simulink model "sm_forklift"  (R2021b)
settings: Solver=ode15s  StartTime=0.0  StopTime=53  MaxStep=1e-2  RelTol=1e-3  AbsTol=1e-3  EnableMultiTasking=on
model workspace: external: MATLAB File sm_forklift_parameters.m (data not in the file)
values from neighbouring files (symbols this model uses):
  g = 9.8    [sm_forklift_parameters.m]
undefined symbols (not defined in the file or in its folder): backRest, box, bump, chassis, fork, infPlane, main_mast, pulley, smiData, tire, top_mast, wheel, X, Y, Z
libraries: sm_lib x1413, nesl_utility x83, fl_lib x23, sm_backhoe_lib x6, SignalEditorBlockLib x1
(part 10 of 24)

== system sm_forklift/Warehouse/Racks/Rack 2/Rack End  ==
  Rack_AngleBrace_21_RIGID : Subsystem
  Rack_AngleBrace_22_RIGID : Subsystem
  Rack_AngleBrace_23_RIGID : Subsystem
  Rack_AngleBrace_24_RIGID : Subsystem
  Rack_AngleBrace_25_RIGID : Subsystem
  Rack_Leg_10_RIGID : Subsystem
  Rack_Leg_9_RIGID : Subsystem
  Rack_ShelfEnd_29_RIGID : Subsystem
  Rack_ShelfEnd_30_RIGID : Subsystem
  Rack_ShelfEnd_31_RIGID : Subsystem
  Rack_ShelfEnd_32_RIGID : Subsystem
  Rack_ShelfEnd_33_RIGID : Subsystem
  Rack_ShelfEnd_34_RIGID : Subsystem
  Rack_ShelfEnd_35_RIGID : Subsystem
  Conn1 : PMIOPort  Side=Left
  connections:
  Conn1/RConn1 -- Rack_ShelfEnd_29_RIGID/LConn2
  Rack_Leg_10_RIGID/LConn1 -- Rack_AngleBrace_25_RIGID/LConn1 -- Rack_AngleBrace_24_RIGID/LConn1 -- Rack_AngleBrace_23_RIGID/LConn1 -- Rack_AngleBrace_22_RIGID/LConn1 -- Rack_ShelfEnd_35_RIGID/LConn1 -- Rack_ShelfEnd_34_RIGID/LConn1 -- Rack_ShelfEnd_33_RIGID/LConn1 -- Rack_ShelfEnd_32_RIGID/LConn1 -- Rack_ShelfEnd_31_RIGID/LConn1 -- Rack_ShelfEnd_29_RIGID/LConn1 -- Rack_AngleBrace_21_RIGID/LConn1 -- Rack_ShelfEnd_30_RIGID/LConn1 -- Rack_Leg_9_RIGID/LConn1

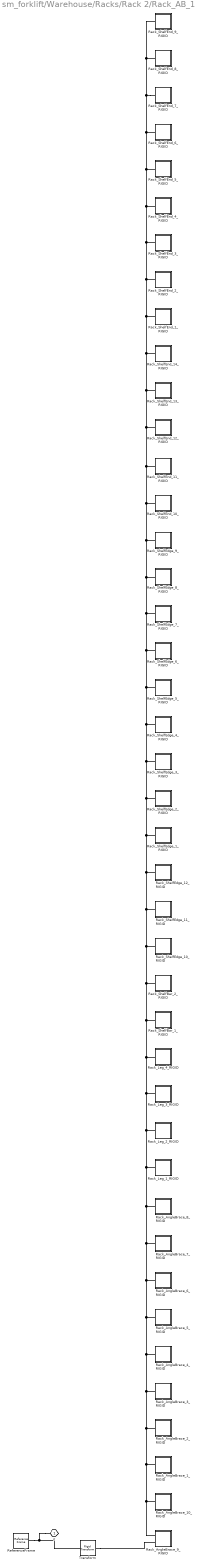
== system sm_forklift/Warehouse/Racks/Rack 2/Rack_AB_1 ==
  Rack_AngleBrace_10_RIGID : Subsystem
  Rack_AngleBrace_1_RIGID : Subsystem
  Rack_AngleBrace_2_RIGID : Subsystem
  Rack_AngleBrace_3_RIGID : Subsystem
  Rack_AngleBrace_4_RIGID : Subsystem
  Rack_AngleBrace_5_RIGID : Subsystem
  Rack_AngleBrace_6_RIGID : Subsystem
  Rack_AngleBrace_7_RIGID : Subsystem
  Rack_AngleBrace_8_RIGID : Subsystem
  Rack_AngleBrace_9_RIGID : Subsystem
  Rack_Leg_1_RIGID : Subsystem
  Rack_Leg_2_RIGID : Subsystem
  Rack_Leg_3_RIGID : Subsystem
  Rack_Leg_4_RIGID : Subsystem
  Rack_ShelfBar_1_RIGID : Subsystem
  Rack_ShelfBar_2_RIGID : Subsystem
  Rack_ShelfEdge_10_RIGID : Subsystem
  Rack_ShelfEdge_11_RIGID : Subsystem
  Rack_ShelfEdge_12_RIGID : Subsystem
  Rack_ShelfEdge_1_RIGID : Subsystem
  Rack_ShelfEdge_2_RIGID : Subsystem
  Rack_ShelfEdge_3_RIGID : Subsystem
  Rack_ShelfEdge_4_RIGID : Subsystem
  Rack_ShelfEdge_5_RIGID : Subsystem
  Rack_ShelfEdge_6_RIGID : Subsystem
  Rack_ShelfEdge_7_RIGID : Subsystem
  Rack_ShelfEdge_8_RIGID : Subsystem
  Rack_ShelfEdge_9_RIGID : Subsystem
  Rack_ShelfEnd_10_RIGID : Subsystem
  Rack_ShelfEnd_11_RIGID : Subsystem
  Rack_ShelfEnd_12_RIGID : Subsystem
  Rack_ShelfEnd_13_RIGID : Subsystem
  Rack_ShelfEnd_14_RIGID : Subsystem
  Rack_ShelfEnd_1_RIGID : Subsystem
  Rack_ShelfEnd_2_RIGID : Subsystem
  Rack_ShelfEnd_3_RIGID : Subsystem
  Rack_ShelfEnd_4_RIGID : Subsystem
  Rack_ShelfEnd_5_RIGID : Subsystem
  Rack_ShelfEnd_6_RIGID : Subsystem
  Rack_ShelfEnd_7_RIGID : Subsystem
  Rack_ShelfEnd_8_RIGID : Subsystem
  Rack_ShelfEnd_9_RIGID : Subsystem
  ReferenceFrame : sm_lib/Frames and Transforms/Reference Frame
  Transform : sm_lib/Frames and Transforms/Rigid Transform  TranslationMethod=Cartesian  TranslationStandardOffset=0  TranslationLengthUnit=m  TranslationStandardAxis=+Z  TranslationCartesianOffset=smiData.RigidTransform(197).translation  TranslationROffset=0  TranslationROffsetUnits=m  TranslationZOffset=0  TranslationZOffsetUnits=m  TranslationThetaOffset=0  TranslationThetaOffsetUnits=deg  RotationMethod=ArbitraryAxis  RotationAngleUnits=rad  RotationStandardAxis=+Z  RotationAngle=smiData.RigidTransform(197).angle  RotationArbitraryAxis=smiData.RigidTransform(197).axis  FollAlignAxisA=+X  BaseAlignAxisA=+Y  FollAlignAxisB=+Y  BaseAlignAxisB=+Z  RotationSequenceAxes=FollowerAxes  RotationSequence=XYX  RotationSequenceAngles=[0 0 0]  RotationSequenceAnglesUnits=deg  RotationMatrix=[1 0 0; 0 1 0; 0 0 1]
  F : PMIOPort  Side=Left
  connections:
  F/RConn1 -- Transform/LConn1 -- ReferenceFrame/RConn1
  Transform/RConn1 -- Rack_AngleBrace_9_RIGID/LConn2
  Rack_ShelfEnd_7_RIGID/LConn1 -- Rack_ShelfEnd_6_RIGID/LConn1 -- Rack_ShelfEnd_5_RIGID/LConn1 -- Rack_ShelfEnd_4_RIGID/LConn1 -- Rack_ShelfEnd_3_RIGID/LConn1 -- Rack_ShelfEnd_2_RIGID/LConn1 -- Rack_ShelfEnd_1_RIGID/LConn1 -- Rack_ShelfEnd_14_RIGID/LConn1 -- Rack_ShelfEnd_13_RIGID/LConn1 -- Rack_ShelfEnd_12_RIGID/LConn1 -- Rack_ShelfEnd_11_RIGID/LConn1 -- Rack_ShelfEnd_10_RIGID/LConn1 -- Rack_ShelfEdge_9_RIGID/LConn1 -- Rack_ShelfEdge_8_RIGID/LConn1 -- Rack_ShelfEdge_7_RIGID/LConn1 -- Rack_ShelfEdge_6_RIGID/LConn1 -- Rack_ShelfEdge_5_RIGID/LConn1 -- Rack_ShelfEdge_4_RIGID/LConn1 -- Rack_ShelfEdge_3_RIGID/LConn1 -- Rack_ShelfEdge_2_RIGID/LConn1 -- Rack_ShelfEdge_1_RIGID/LConn1 -- Rack_ShelfEdge_12_RIGID/LConn1 -- Rack_ShelfEdge_11_RIGID/LConn1 -- Rack_ShelfEdge_10_RIGID/LConn1 -- Rack_ShelfBar_2_RIGID/LConn1 -- Rack_ShelfBar_1_RIGID/LConn1 -- Rack_Leg_4_RIGID/LConn1 -- Rack_Leg_3_RIGID/LConn1 -- Rack_Leg_2_RIGID/LConn1 -- Rack_Leg_1_RIGID/LConn1 -- Rack_AngleBrace_8_RIGID/LConn1 -- Rack_AngleBrace_7_RIGID/LConn1 -- Rack_AngleBrace_6_RIGID/LConn1 -- Rack_AngleBrace_5_RIGID/LConn1 -- Rack_AngleBrace_4_RIGID/LConn1 -- Rack_AngleBrace_3_RIGID/LConn1 -- Rack_AngleBrace_2_RIGID/LConn1 -- Rack_AngleBrace_1_RIGID/LConn1 -- Rack_AngleBrace_9_RIGID/LConn1 -- Rack_AngleBrace_10_RIGID/LConn1 -- Rack_ShelfEnd_9_RIGID/LConn1 -- Rack_ShelfEnd_8_RIGID/LConn1

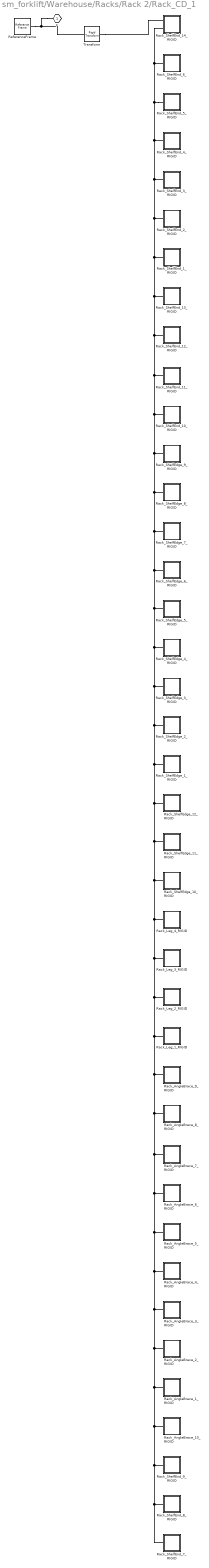
== system sm_forklift/Warehouse/Racks/Rack 2/Rack_CD_1 ==
  Rack_AngleBrace_10_RIGID : Subsystem
  Rack_AngleBrace_1_RIGID : Subsystem
  Rack_AngleBrace_2_RIGID : Subsystem
  Rack_AngleBrace_3_RIGID : Subsystem
  Rack_AngleBrace_4_RIGID : Subsystem
  Rack_AngleBrace_5_RIGID : Subsystem
  Rack_AngleBrace_6_RIGID : Subsystem
  Rack_AngleBrace_7_RIGID : Subsystem
  Rack_AngleBrace_8_RIGID : Subsystem
  Rack_AngleBrace_9_RIGID : Subsystem
  Rack_Leg_1_RIGID : Subsystem
  Rack_Leg_2_RIGID : Subsystem
  Rack_Leg_3_RIGID : Subsystem
  Rack_Leg_4_RIGID : Subsystem
  Rack_ShelfEdge_10_RIGID : Subsystem
  Rack_ShelfEdge_11_RIGID : Subsystem
  Rack_ShelfEdge_12_RIGID : Subsystem
  Rack_ShelfEdge_1_RIGID : Subsystem
  Rack_ShelfEdge_2_RIGID : Subsystem
  Rack_ShelfEdge_3_RIGID : Subsystem
  Rack_ShelfEdge_4_RIGID : Subsystem
  Rack_ShelfEdge_5_RIGID : Subsystem
  Rack_ShelfEdge_6_RIGID : Subsystem
  Rack_ShelfEdge_7_RIGID : Subsystem
  Rack_ShelfEdge_8_RIGID : Subsystem
  Rack_ShelfEdge_9_RIGID : Subsystem
  Rack_ShelfEnd_10_RIGID : Subsystem
  Rack_ShelfEnd_11_RIGID : Subsystem
  Rack_ShelfEnd_12_RIGID : Subsystem
  Rack_ShelfEnd_13_RIGID : Subsystem
  Rack_ShelfEnd_14_RIGID : Subsystem
  Rack_ShelfEnd_1_RIGID : Subsystem
  Rack_ShelfEnd_2_RIGID : Subsystem
  Rack_ShelfEnd_3_RIGID : Subsystem
  Rack_ShelfEnd_4_RIGID : Subsystem
  Rack_ShelfEnd_5_RIGID : Subsystem
  Rack_ShelfEnd_6_RIGID : Subsystem
  Rack_ShelfEnd_7_RIGID : Subsystem
  Rack_ShelfEnd_8_RIGID : Subsystem
  Rack_ShelfEnd_9_RIGID : Subsystem
  ReferenceFrame : sm_lib/Frames and Transforms/Reference Frame
  Transform : sm_lib/Frames and Transforms/Rigid Transform  TranslationMethod=Cartesian  TranslationStandardOffset=0  TranslationLengthUnit=m  TranslationStandardAxis=+Z  TranslationCartesianOffset=smiData.RigidTransform(193).translation  TranslationROffset=0  TranslationROffsetUnits=m  TranslationZOffset=0  TranslationZOffsetUnits=m  TranslationThetaOffset=0  TranslationThetaOffsetUnits=deg  RotationMethod=ArbitraryAxis  RotationAngleUnits=rad  RotationStandardAxis=+Z  RotationAngle=smiData.RigidTransform(193).angle  RotationArbitraryAxis=smiData.RigidTransform(193).axis  FollAlignAxisA=+X  BaseAlignAxisA=+Y  FollAlignAxisB=+Y  BaseAlignAxisB=+Z  RotationSequenceAxes=FollowerAxes  RotationSequence=XYX  RotationSequenceAngles=[0 0 0]  RotationSequenceAnglesUnits=deg  RotationMatrix=[1 0 0; 0 1 0; 0 0 1]
  F : PMIOPort  Side=Left
  connections:
  F/RConn1 -- Transform/LConn1 -- ReferenceFrame/RConn1
  Transform/RConn1 -- Rack_ShelfEnd_14_RIGID/LConn1
  Rack_ShelfEnd_5_RIGID/LConn1 -- Rack_ShelfEnd_4_RIGID/LConn1 -- Rack_ShelfEnd_3_RIGID/LConn1 -- Rack_ShelfEnd_2_RIGID/LConn1 -- Rack_ShelfEnd_1_RIGID/LConn1 -- Rack_ShelfEnd_13_RIGID/LConn1 -- Rack_ShelfEnd_12_RIGID/LConn1 -- Rack_ShelfEnd_11_RIGID/LConn1 -- Rack_ShelfEnd_10_RIGID/LConn1 -- Rack_ShelfEdge_9_RIGID/LConn1 -- Rack_ShelfEdge_8_RIGID/LConn1 -- Rack_ShelfEdge_7_RIGID/LConn1 -- Rack_ShelfEdge_6_RIGID/LConn1 -- Rack_ShelfEdge_5_RIGID/LConn1 -- Rack_ShelfEdge_4_RIGID/LConn1 -- Rack_ShelfEdge_3_RIGID/LConn1 -- Rack_ShelfEdge_2_RIGID/LConn1 -- Rack_ShelfEdge_1_RIGID/LConn1 -- Rack_ShelfEdge_12_RIGID/LConn1 -- Rack_ShelfEdge_11_RIGID/LConn1 -- Rack_ShelfEdge_10_RIGID/LConn1 -- Rack_Leg_4_RIGID/LConn1 -- Rack_Leg_3_RIGID/LConn1 -- Rack_Leg_2_RIGID/LConn1 -- Rack_Leg_1_RIGID/LConn1 -- Rack_AngleBrace_9_RIGID/LConn1 -- Rack_AngleBrace_8_RIGID/LConn1 -- Rack_AngleBrace_7_RIGID/LConn1 -- Rack_AngleBrace_6_RIGID/LConn1 -- Rack_AngleBrace_5_RIGID/LConn1 -- Rack_AngleBrace_4_RIGID/LConn1 -- Rack_AngleBrace_3_RIGID/LConn1 -- Rack_AngleBrace_2_RIGID/LConn1 -- Rack_AngleBrace_1_RIGID/LConn1 -- Rack_ShelfEnd_9_RIGID/LConn1 -- Rack_ShelfEnd_8_RIGID/LConn1 -- Rack_ShelfEnd_7_RIGID/LConn1 -- Rack_AngleBrace_10_RIGID/LConn1 -- Rack_ShelfEnd_6_RIGID/LConn1 -- Rack_ShelfEnd_14_RIGID/LConn2

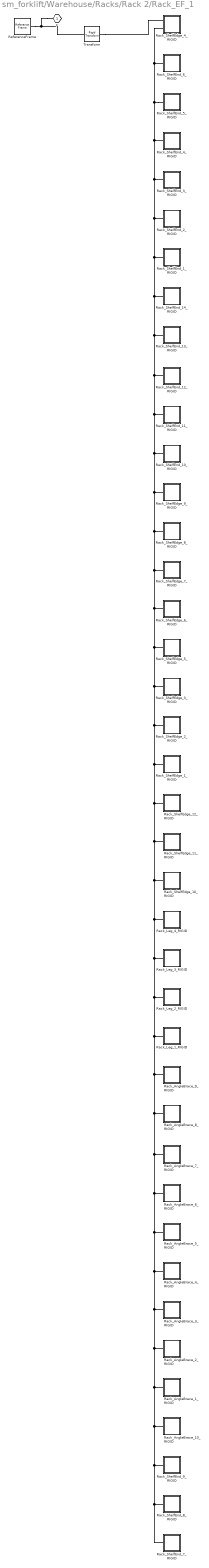
== system sm_forklift/Warehouse/Racks/Rack 2/Rack_EF_1 ==
  Rack_AngleBrace_10_RIGID : Subsystem
  Rack_AngleBrace_1_RIGID : Subsystem
  Rack_AngleBrace_2_RIGID : Subsystem
  Rack_AngleBrace_3_RIGID : Subsystem
  Rack_AngleBrace_4_RIGID : Subsystem
  Rack_AngleBrace_5_RIGID : Subsystem
  Rack_AngleBrace_6_RIGID : Subsystem
  Rack_AngleBrace_7_RIGID : Subsystem
  Rack_AngleBrace_8_RIGID : Subsystem
  Rack_AngleBrace_9_RIGID : Subsystem
  Rack_Leg_1_RIGID : Subsystem
  Rack_Leg_2_RIGID : Subsystem
  Rack_Leg_3_RIGID : Subsystem
  Rack_Leg_4_RIGID : Subsystem
  Rack_ShelfEdge_10_RIGID : Subsystem
  Rack_ShelfEdge_11_RIGID : Subsystem
  Rack_ShelfEdge_12_RIGID : Subsystem
  Rack_ShelfEdge_1_RIGID : Subsystem
  Rack_ShelfEdge_2_RIGID : Subsystem
  Rack_ShelfEdge_3_RIGID : Subsystem
  Rack_ShelfEdge_4_RIGID : Subsystem
  Rack_ShelfEdge_5_RIGID : Subsystem
  Rack_ShelfEdge_6_RIGID : Subsystem
  Rack_ShelfEdge_7_RIGID : Subsystem
  Rack_ShelfEdge_8_RIGID : Subsystem
  Rack_ShelfEdge_9_RIGID : Subsystem
  Rack_ShelfEnd_10_RIGID : Subsystem
  Rack_ShelfEnd_11_RIGID : Subsystem
  Rack_ShelfEnd_12_RIGID : Subsystem
  Rack_ShelfEnd_13_RIGID : Subsystem
  Rack_ShelfEnd_14_RIGID : Subsystem
  Rack_ShelfEnd_1_RIGID : Subsystem
  Rack_ShelfEnd_2_RIGID : Subsystem
  Rack_ShelfEnd_3_RIGID : Subsystem
  Rack_ShelfEnd_4_RIGID : Subsystem
  Rack_ShelfEnd_5_RIGID : Subsystem
  Rack_ShelfEnd_6_RIGID : Subsystem
  Rack_ShelfEnd_7_RIGID : Subsystem
  Rack_ShelfEnd_8_RIGID : Subsystem
  Rack_ShelfEnd_9_RIGID : Subsystem
  ReferenceFrame : sm_lib/Frames and Transforms/Reference Frame
  Transform : sm_lib/Frames and Transforms/Rigid Transform  TranslationMethod=Cartesian  TranslationStandardOffset=0  TranslationLengthUnit=m  TranslationStandardAxis=+Z  TranslationCartesianOffset=smiData.RigidTransform(195).translation  TranslationROffset=0  TranslationROffsetUnits=m  TranslationZOffset=0  TranslationZOffsetUnits=m  TranslationThetaOffset=0  TranslationThetaOffsetUnits=deg  RotationMethod=ArbitraryAxis  RotationAngleUnits=rad  RotationStandardAxis=+Z  RotationAngle=smiData.RigidTransform(195).angle  RotationArbitraryAxis=smiData.RigidTransform(195).axis  FollAlignAxisA=+X  BaseAlignAxisA=+Y  FollAlignAxisB=+Y  BaseAlignAxisB=+Z  RotationSequenceAxes=FollowerAxes  RotationSequence=XYX  RotationSequenceAngles=[0 0 0]  RotationSequenceAnglesUnits=deg  RotationMatrix=[1 0 0; 0 1 0; 0 0 1]
  F : PMIOPort  Side=Left
  connections:
  F/RConn1 -- Transform/LConn1 -- ReferenceFrame/RConn1
  Transform/RConn1 -- Rack_ShelfEdge_4_RIGID/LConn1
  Rack_ShelfEnd_5_RIGID/LConn1 -- Rack_ShelfEnd_4_RIGID/LConn1 -- Rack_ShelfEnd_3_RIGID/LConn1 -- Rack_ShelfEnd_2_RIGID/LConn1 -- Rack_ShelfEnd_1_RIGID/LConn1 -- Rack_ShelfEnd_14_RIGID/LConn1 -- Rack_ShelfEnd_13_RIGID/LConn1 -- Rack_ShelfEnd_12_RIGID/LConn1 -- Rack_ShelfEnd_11_RIGID/LConn1 -- Rack_ShelfEnd_10_RIGID/LConn1 -- Rack_ShelfEdge_9_RIGID/LConn1 -- Rack_ShelfEdge_8_RIGID/LConn1 -- Rack_ShelfEdge_7_RIGID/LConn1 -- Rack_ShelfEdge_6_RIGID/LConn1 -- Rack_ShelfEdge_5_RIGID/LConn1 -- Rack_ShelfEdge_3_RIGID/LConn1 -- Rack_ShelfEdge_2_RIGID/LConn1 -- Rack_ShelfEdge_1_RIGID/LConn1 -- Rack_ShelfEdge_12_RIGID/LConn1 -- Rack_ShelfEdge_11_RIGID/LConn1 -- Rack_ShelfEdge_10_RIGID/LConn1 -- Rack_Leg_4_RIGID/LConn1 -- Rack_Leg_3_RIGID/LConn1 -- Rack_Leg_2_RIGID/LConn1 -- Rack_Leg_1_RIGID/LConn1 -- Rack_AngleBrace_9_RIGID/LConn1 -- Rack_AngleBrace_8_RIGID/LConn1 -- Rack_AngleBrace_7_RIGID/LConn1 -- Rack_AngleBrace_6_RIGID/LConn1 -- Rack_AngleBrace_5_RIGID/LConn1 -- Rack_AngleBrace_4_RIGID/LConn1 -- Rack_AngleBrace_3_RIGID/LConn1 -- Rack_AngleBrace_2_RIGID/LConn1 -- Rack_AngleBrace_1_RIGID/LConn1 -- Rack_ShelfEnd_9_RIGID/LConn1 -- Rack_ShelfEnd_8_RIGID/LConn1 -- Rack_ShelfEnd_7_RIGID/LConn1 -- Rack_AngleBrace_10_RIGID/LConn1 -- Rack_ShelfEnd_6_RIGID/LConn1 -- Rack_ShelfEdge_4_RIGID/LConn2

== system sm_forklift/Forklift/Masts/Lift Mechanism/Left Lift Cylinder/Cylinder Assembly ==
  Base to Cylinder Transform : sm_lib/Frames and Transforms/Rigid Transform  TranslationMethod=StandardAxis  TranslationStandardOffset=(Lcyl/2)  TranslationLengthUnit=m  TranslationStandardAxis=-Z  TranslationCartesianOffset=[0 0 0]  TranslationROffset=0  TranslationROffsetUnits=m  TranslationZOffset=0  TranslationZOffsetUnits=m  TranslationThetaOffset=0  TranslationThetaOffsetUnits=deg  RotationMethod=AlignedAxes  RotationAngleUnits=deg  RotationStandardAxis=+X  RotationAngle=90  RotationArbitraryAxis=[0 0 1]  FollAlignAxisA=+X  BaseAlignAxisA=+X  FollAlignAxisB=+Z  BaseAlignAxisB=-Z  RotationSequenceAxes=FollowerAxes  RotationSequence=XYX  RotationSequenceAngles=[0 0 0]  RotationSequenceAnglesUnits=deg  RotationMatrix=[1 0 0; 0 1 0; 0 0 1]
  Cylinder : sm_lib/Body Elements/Extruded Solid  GraphicAmbientColor=[0.15 0.15 0.15 1.0]  BasedOnType=Density  CenterOfMass=[0 0 0]  CenterOfMassUnits=m  GraphicDiffuseColor=cylColor  ExportConvexHullGeometry=off  ExtrusionCrossSection=cylSection  ExtrusionCrossSectionUnits=m  Density=rhoCyl  DensityUnits=kg/(m^3)  DoExposeReferenceFrame=on  GraphicEmissiveColor=[0.0 0.0 0.0 1.0]  ExportEntireGeometry=off  ExtrusionLength=Lcyl  ExtrusionLengthUnits=m  ExtrusionType=General  SerializedFrames=<Frames/>  MarkerShape=Sphere  MarkerSize=10  GraphicType=FromGeometry  InertiaType=CalculateFromGeometry  Mass=1  MassUnits=kg  MomentsOfInertia=[1 1 1]  MomentsOfInertiaUnits=kg*m^2  PolygonNumSides=3  GraphicOpacity=1.0  PolygonOuterRadius=1  PolygonOuterRadiusUnits=m  ProductsOfInertia=[0 0 0]  ProductsOfInertiaUnits=kg*m^2  GraphicShininess=75  GraphicSpecularColor=[0.5 0.5 0.5 1.0]  GraphicVisPropType=SimpleVisualProperties
  Single Bracket : sm_backhoe_lib/Single Bracket  Hbracket=Lbase  Wbracket=Wbase  Tbracket=0.03  Hhole=Lbase-(Wbase/2)  Rhole=Rbp  Nc=circlePointsCylB  bracketColor=connColor  rho=rhoConn
      settings: SourceProductBaseCode=MS
  Base Hole : PMIOPort  Side=Right
  Prismatic : PMIOPort  Port=2  Side=Left
  connections:
  Single Bracket/RConn1 -- Base Hole/RConn1
  Single Bracket/LConn1 -- Base to Cylinder Transform/RConn1
  Cylinder/RConn1 -- Base to Cylinder Transform/LConn1 -- Prismatic/RConn1

== system sm_forklift/Forklift/Masts/Lift Mechanism/Left Lift Cylinder/Piston Assembly ==
  Piston : sm_lib/Body Elements/Cylindrical Solid  GraphicAmbientColor=[0.15 0.15 0.15 1.0]  BasedOnType=Density  CenterOfMass=[0 0 0]  CenterOfMassUnits=m  GraphicDiffuseColor=pistColor  CylinderLength=Lpist  CylinderLengthUnits=m  CylinderRadius=Rpist  CylinderRadiusUnits=m  Density=rhoPist  DensityUnits=kg/(m^3)  DoExposeReferenceFrame=on  GraphicEmissiveColor=[0.0 0.0 0.0 1.0]  ExportEntireGeometry=off  SerializedFrames=<Frames/>  MarkerShape=Sphere  MarkerSize=10  GraphicType=FromGeometry  InertiaType=CalculateFromGeometry  Mass=1  MassUnits=kg  MomentsOfInertia=[1 1 1]  MomentsOfInertiaUnits=kg*m^2  GraphicOpacity=1.0  ProductsOfInertia=[0 0 0]  ProductsOfInertiaUnits=kg*m^2  GraphicShininess=75  GraphicSpecularColor=[0.5 0.5 0.5 1.0]  GraphicVisPropType=SimpleVisualProperties
  Piston to Head Transform : sm_lib/Frames and Transforms/Rigid Transform  TranslationMethod=StandardAxis  TranslationStandardOffset=Lpist/2  TranslationLengthUnit=m  TranslationStandardAxis=+Z  TranslationCartesianOffset=[0 0 0]  TranslationROffset=0  TranslationROffsetUnits=m  TranslationZOffset=0  TranslationZOffsetUnits=m  TranslationThetaOffset=0  TranslationThetaOffsetUnits=deg  RotationMethod=AlignedAxes  RotationAngleUnits=deg  RotationStandardAxis=-X  RotationAngle=90  RotationArbitraryAxis=[0 0 1]  FollAlignAxisA=+Y  BaseAlignAxisA=-Y  FollAlignAxisB=+Z  BaseAlignAxisB=+Z  RotationSequenceAxes=FollowerAxes  RotationSequence=XYX  RotationSequenceAngles=[0 0 0]  RotationSequenceAnglesUnits=deg  RotationMatrix=[1 0 0; 0 1 0; 0 0 1]
  Prismatic : PMIOPort  Side=Left
  Head Hole : PMIOPort  Port=2  Side=Right
  connections:
  Piston to Head Transform/RConn1 -- Head Hole/RConn1
  Prismatic/RConn1 -- Piston to Head Transform/LConn1 -- Piston/RConn1

== system sm_forklift/Forklift/Masts/Lift Mechanism/Right Lift Cylinder/Cylinder Assembly ==
  Base to Cylinder Transform : sm_lib/Frames and Transforms/Rigid Transform  TranslationMethod=StandardAxis  TranslationStandardOffset=(Lcyl/2)  TranslationLengthUnit=m  TranslationStandardAxis=-Z  TranslationCartesianOffset=[0 0 0]  TranslationROffset=0  TranslationROffsetUnits=m  TranslationZOffset=0  TranslationZOffsetUnits=m  TranslationThetaOffset=0  TranslationThetaOffsetUnits=deg  RotationMethod=AlignedAxes  RotationAngleUnits=deg  RotationStandardAxis=+X  RotationAngle=90  RotationArbitraryAxis=[0 0 1]  FollAlignAxisA=+X  BaseAlignAxisA=+X  FollAlignAxisB=+Z  BaseAlignAxisB=-Z  RotationSequenceAxes=FollowerAxes  RotationSequence=XYX  RotationSequenceAngles=[0 0 0]  RotationSequenceAnglesUnits=deg  RotationMatrix=[1 0 0; 0 1 0; 0 0 1]
  Cylinder : sm_lib/Body Elements/Extruded Solid  GraphicAmbientColor=[0.15 0.15 0.15 1.0]  BasedOnType=Density  CenterOfMass=[0 0 0]  CenterOfMassUnits=m  GraphicDiffuseColor=cylColor  ExportConvexHullGeometry=off  ExtrusionCrossSection=cylSection  ExtrusionCrossSectionUnits=m  Density=rhoCyl  DensityUnits=kg/(m^3)  DoExposeReferenceFrame=on  GraphicEmissiveColor=[0.0 0.0 0.0 1.0]  ExportEntireGeometry=off  ExtrusionLength=Lcyl  ExtrusionLengthUnits=m  ExtrusionType=General  SerializedFrames=<Frames/>  MarkerShape=Sphere  MarkerSize=10  GraphicType=FromGeometry  InertiaType=CalculateFromGeometry  Mass=1  MassUnits=kg  MomentsOfInertia=[1 1 1]  MomentsOfInertiaUnits=kg*m^2  PolygonNumSides=3  GraphicOpacity=1.0  PolygonOuterRadius=1  PolygonOuterRadiusUnits=m  ProductsOfInertia=[0 0 0]  ProductsOfInertiaUnits=kg*m^2  GraphicShininess=75  GraphicSpecularColor=[0.5 0.5 0.5 1.0]  GraphicVisPropType=SimpleVisualProperties
  Single Bracket : sm_backhoe_lib/Single Bracket  Hbracket=Lbase  Wbracket=Wbase  Tbracket=0.03  Hhole=Lbase-(Wbase/2)  Rhole=Rbp  Nc=circlePointsCylB  bracketColor=connColor  rho=rhoConn
      settings: SourceProductBaseCode=MS
  Base Hole : PMIOPort  Side=Right
  Prismatic : PMIOPort  Port=2  Side=Left
  connections:
  Prismatic/RConn1 -- Base to Cylinder Transform/LConn1 -- Cylinder/RConn1
  Single Bracket/LConn1 -- Base to Cylinder Transform/RConn1
  Single Bracket/RConn1 -- Base Hole/RConn1

== system sm_forklift/Forklift/Masts/Lift Mechanism/Right Lift Cylinder/Hydraulic Actuator ==
  Pressure Input : Inport
  Add : Sum
  Add1 : Sum  Inputs=+-
  Custom Hydraulic Fluid : fl_lib/Hydraulic/Hydraulic Utilities/Custom Hydraulic Fluid  density=850 kg/m^3  viscosity_kin=18e-6 m^2/s  bulk=0.8e9 Pa  alpha=0.005  range_error=2
      settings: SourceProductBaseCode=SS  InternalSimscapePortConfiguration="{\"Bottom\":[],\"Left\":[],\"Right\":[{\"id\":\"G\",\"label\":\"\",\"type\":\"foundation.hydraulic.hydraulic\"}],\"Top\":[]}"
  Cylinder Side Chamber : fl_lib/Hydraulic/Hydraulic Elements/Translational Hydro-Mechanical Converter  area=pi*(Rcyl^2) m^2  or=1  compressibility=0  displacement_spec=foundation.enum.DisplacementSpec.Calculate  init_pos=0 m  V_dead=1e-4 m^3  k_sh=1.4  initial_pressure=0 Pa
      settings: SourceProductBaseCode=SS  InternalSimscapePortConfiguration="{\"Bottom\":[],\"Left\":[{\"id\":\"C\",\"label\":\"C\",\"type\":\"foundation.mechanical.translational.translational\"},{\"id\":\"A\",\"label\":\"A\",\"type\":\"foundation.hydraulic.hydraulic\"}],\"Right\":[{\"id\":\"R\",\"label\":\"R\",\"type\":\"foundation.mechanical.translational.translational\"}],\"Top\":[]}"
  Gain : Gain  Gain=1/2
  Gain1 : Gain  Gain=1/2
  Hydraulic Reference : fl_lib/Hydraulic/Hydraulic Elements/Hydraulic Reference
  Linear Hydraulic Resistance : fl_lib/Hydraulic/Hydraulic Elements/Linear Hydraulic Resistance  resistance=1e5 Pa/(m^3/s)  q_specify=off  q_priority=None  q=0.001 m^3/s  q_nominal_specify=off  q_nominal_unit=m^3/s  q_nominal_value=1  p_specify=off  p_priority=None  p=0 Pa  p_nominal_specify=off  p_nominal_unit=Pa  p_nominal_value=1
      settings: SourceProductBaseCode=SS  InternalSimscapePortConfiguration="{\"Bottom\":[],\"Left\":[{\"id\":\"A\",\"label\":\"A\",\"type\":\"foundation.hydraulic.hydraulic\"}],\"Right\":[{\"id\":\"B\",\"label\":\"B\",\"type\":\"foundation.hydraulic.hydraulic\"}],\"Top\":[]}"
  Linear Hydraulic Resistance1 : fl_lib/Hydraulic/Hydraulic Elements/Linear Hydraulic Resistance  resistance=1e5 Pa/(m^3/s)  q_specify=off  q_priority=None  q=0.001 m^3/s  q_nominal_specify=off  q_nominal_unit=m^3/s  q_nominal_value=1  p_specify=off  p_priority=None  p=0 Pa  p_nominal_specify=off  p_nominal_unit=Pa  p_nominal_value=1
      settings: SourceProductBaseCode=SS  InternalSimscapePortConfiguration="{\"Bottom\":[],\"Left\":[{\"id\":\"A\",\"label\":\"A\",\"type\":\"foundation.hydraulic.hydraulic\"}],\"Right\":[{\"id\":\"B\",\"label\":\"B\",\"type\":\"foundation.hydraulic.hydraulic\"}],\"Top\":[]}"
  Mechanical Translational Reference : fl_lib/Mechanical/Translational Elements/Mechanical Translational Reference
  Nominal Pressure : Constant  Value=350
  Piston Head Side Chamber : fl_lib/Hydraulic/Hydraulic Elements/Translational Hydro-Mechanical Converter  area=pi*(Rcyl^2) m^2  or=2  compressibility=0  displacement_spec=foundation.enum.DisplacementSpec.Calculate  init_pos=0 m  V_dead=1e-4 m^3  k_sh=1.4  initial_pressure=0 Pa
      settings: SourceProductBaseCode=SS  InternalSimscapePortConfiguration="{\"Bottom\":[],\"Left\":[{\"id\":\"C\",\"label\":\"C\",\"type\":\"foundation.mechanical.translational.translational\"},{\"id\":\"A\",\"label\":\"A\",\"type\":\"foundation.hydraulic.hydraulic\"}],\"Right\":[{\"id\":\"R\",\"label\":\"R\",\"type\":\"foundation.mechanical.translational.translational\"}],\"Top\":[]}"
  Pressure Difference : fl_lib/Hydraulic/Hydraulic Sources/Hydraulic Pressure Source
      settings: SourceProductBaseCode=SS  InternalSimscapePortConfiguration="{\"Bottom\":[],\"Left\":[{\"id\":\"P\",\"label\":\"P\",\"type\":\"foundation.hydraulic.hydraulic\"}],\"Right\":[{\"id\":\"S\",\"label\":\"S\",\"type\":\"input\"},{\"id\":\"T\",\"label\":\"T\",\"type\":\"foundation.hydraulic.hydraulic\"}],\"Top\":[]}"
  Pressure Difference1 : fl_lib/Hydraulic/Hydraulic Sources/Hydraulic Pressure Source
      settings: SourceProductBaseCode=SS  InternalSimscapePortConfiguration="{\"Bottom\":[],\"Left\":[{\"id\":\"P\",\"label\":\"P\",\"type\":\"foundation.hydraulic.hydraulic\"}],\"Right\":[{\"id\":\"S\",\"label\":\"S\",\"type\":\"input\"},{\"id\":\"T\",\"label\":\"T\",\"type\":\"foundation.hydraulic.hydraulic\"}],\"Top\":[]}"
  Simulink-PS Converter : nesl_utility/Simulink-PS Converter  PhysicalDomain=network_engine_domain  SubClassName=ps_input  LeftPortType=input  RightPortType=output  PseudoPeriodic=off  Frequencies=[]  NoiseDistribution=none  NoiseParameters=[]  Unit=bar  AffineConversion=off  FilteringAndDerivatives=filter  SimscapeFilterOrder=1  InputFilterTimeConstant=.001  UdotUserProvided=1
      settings: SourceProductBaseCode=PW,SS
  Simulink-PS Converter1 : nesl_utility/Simulink-PS Converter  PhysicalDomain=network_engine_domain  SubClassName=ps_input  LeftPortType=input  RightPortType=output  PseudoPeriodic=off  Frequencies=[]  NoiseDistribution=none  NoiseParameters=[]  Unit=bar  AffineConversion=off  FilteringAndDerivatives=filter  SimscapeFilterOrder=1  InputFilterTimeConstant=.001  UdotUserProvided=1
      settings: SourceProductBaseCode=PW,SS
  R : PMIOPort  Side=Right
  C : PMIOPort  Port=2  Side=Right
  wires:
  Pressure Input/1 -> Gain/1, Gain1/1
  Nominal Pressure/1 -> Add/2, Add1/1
  Gain/1 -> Add/1
  Add/1 -> Simulink-PS Converter/1
  Add1/1 -> Simulink-PS Converter1/1
  Gain1/1 -> Add1/2
  connections:
  Mechanical Translational Reference/LConn1 -- Piston Head Side Chamber/LConn1 -- C/RConn1 -- Cylinder Side Chamber/LConn1
  Cylinder Side Chamber/RConn1 -- Piston Head Side Chamber/RConn1 -- R/RConn1
  Custom Hydraulic Fluid/RConn1 -- Linear Hydraulic Resistance/LConn1 -- Pressure Difference/LConn1
  Hydraulic Reference/LConn1 -- Pressure Difference/RConn2 -- Pressure Difference1/RConn2
  Simulink-PS Converter/RConn1 -- Pressure Difference/RConn1
  Simulink-PS Converter1/RConn1 -- Pressure Difference1/RConn1
  Linear Hydraulic Resistance/RConn1 -- Cylinder Side Chamber/LConn2
  Linear Hydraulic Resistance1/RConn1 -- Piston Head Side Chamber/LConn2
  Linear Hydraulic Resistance1/LConn1 -- Pressure Difference1/LConn1

== system sm_forklift/Forklift/Masts/Lift Mechanism/Right Lift Cylinder/Piston Assembly ==
  Piston : sm_lib/Body Elements/Cylindrical Solid  GraphicAmbientColor=[0.15 0.15 0.15 1.0]  BasedOnType=Density  CenterOfMass=[0 0 0]  CenterOfMassUnits=m  GraphicDiffuseColor=pistColor  CylinderLength=Lpist  CylinderLengthUnits=m  CylinderRadius=Rpist  CylinderRadiusUnits=m  Density=rhoPist  DensityUnits=kg/(m^3)  DoExposeReferenceFrame=on  GraphicEmissiveColor=[0.0 0.0 0.0 1.0]  ExportEntireGeometry=off  SerializedFrames=<Frames/>  MarkerShape=Sphere  MarkerSize=10  GraphicType=FromGeometry  InertiaType=CalculateFromGeometry  Mass=1  MassUnits=kg  MomentsOfInertia=[1 1 1]  MomentsOfInertiaUnits=kg*m^2  GraphicOpacity=1.0  ProductsOfInertia=[0 0 0]  ProductsOfInertiaUnits=kg*m^2  GraphicShininess=75  GraphicSpecularColor=[0.5 0.5 0.5 1.0]  GraphicVisPropType=SimpleVisualProperties
  Piston to Head Transform : sm_lib/Frames and Transforms/Rigid Transform  TranslationMethod=StandardAxis  TranslationStandardOffset=Lpist/2  TranslationLengthUnit=m  TranslationStandardAxis=+Z  TranslationCartesianOffset=[0 0 0]  TranslationROffset=0  TranslationROffsetUnits=m  TranslationZOffset=0  TranslationZOffsetUnits=m  TranslationThetaOffset=0  TranslationThetaOffsetUnits=deg  RotationMethod=AlignedAxes  RotationAngleUnits=deg  RotationStandardAxis=-X  RotationAngle=90  RotationArbitraryAxis=[0 0 1]  FollAlignAxisA=+Y  BaseAlignAxisA=-Y  FollAlignAxisB=+Z  BaseAlignAxisB=+Z  RotationSequenceAxes=FollowerAxes  RotationSequence=XYX  RotationSequenceAngles=[0 0 0]  RotationSequenceAnglesUnits=deg  RotationMatrix=[1 0 0; 0 1 0; 0 0 1]
  Prismatic : PMIOPort  Side=Left
  Head Hole : PMIOPort  Port=2  Side=Right
  connections:
  Piston/RConn1 -- Piston to Head Transform/LConn1 -- Prismatic/RConn1
  Piston to Head Transform/RConn1 -- Head Hole/RConn1

== system sm_forklift/Forklift/Masts/Lift Mechanism/Right Lift Cylinder/Simscape Interface ==
  Ideal Force Sensor : fl_lib/Mechanical/Mechanical Sensors/Ideal Force Sensor
  Ideal Translational Velocity Source : fl_lib/Mechanical/Mechanical Sources/Ideal Translational Velocity Source
  R : PMIOPort  Side=Right
  C : PMIOPort  Port=2  Side=Right
  F : PMIOPort  Port=3  Side=Left
  V : PMIOPort  Port=4  Side=Left
  connections:
  Ideal Force Sensor/RConn1 -- Ideal Translational Velocity Source/LConn1
  V/RConn1 -- Ideal Translational Velocity Source/RConn1
  C/RConn1 -- Ideal Translational Velocity Source/RConn2
  Ideal Force Sensor/LConn1 -- R/RConn1
  Ideal Force Sensor/RConn2 -- F/RConn1

== system sm_forklift/Forklift/Masts/Tilt Mechanism/Left Tilt Cylinder/Cylinder Assembly ==
  Base to Cylinder Transform : sm_lib/Frames and Transforms/Rigid Transform  TranslationMethod=StandardAxis  TranslationStandardOffset=(Lcyl/2)  TranslationLengthUnit=m  TranslationStandardAxis=-Z  TranslationCartesianOffset=[0 0 0]  TranslationROffset=0  TranslationROffsetUnits=m  TranslationZOffset=0  TranslationZOffsetUnits=m  TranslationThetaOffset=0  TranslationThetaOffsetUnits=deg  RotationMethod=AlignedAxes  RotationAngleUnits=deg  RotationStandardAxis=+X  RotationAngle=90  RotationArbitraryAxis=[0 0 1]  FollAlignAxisA=+X  BaseAlignAxisA=+X  FollAlignAxisB=+Z  BaseAlignAxisB=-Z  RotationSequenceAxes=FollowerAxes  RotationSequence=XYX  RotationSequenceAngles=[0 0 0]  RotationSequenceAnglesUnits=deg  RotationMatrix=[1 0 0; 0 1 0; 0 0 1]
  Cylinder : sm_lib/Body Elements/Extruded Solid  GraphicAmbientColor=[0.15 0.15 0.15 1.0]  BasedOnType=Density  CenterOfMass=[0 0 0]  CenterOfMassUnits=m  GraphicDiffuseColor=cylColor  ExportConvexHullGeometry=off  ExtrusionCrossSection=cylSection  ExtrusionCrossSectionUnits=m  Density=rhoCyl  DensityUnits=kg/(m^3)  DoExposeReferenceFrame=on  GraphicEmissiveColor=[0.0 0.0 0.0 1.0]  ExportEntireGeometry=off  ExtrusionLength=Lcyl  ExtrusionLengthUnits=m  ExtrusionType=General  SerializedFrames=<Frames><Frame><Id>Frame1</Id><Value><Name>F1</Name><Origin><Source>GeometricFeature</Source><FeatureName>top surface</FeatureName></Origin><PrimaryAxis><DefinedDirection>+Z</DefinedDirection><Source>ReferenceFrame</Source><SourceDirection>+Z</SourceDirection><FeatureName></FeatureName></PrimaryAxis><SecondaryAxis><DefinedDirection>+X</DefinedDirection><Source>ReferenceFrame</Source><SourceDirection>+X</SourceDirection><FeatureName></FeatureName></SecondaryAxis></Value></Frame></Frames>  MarkerShape=Sphere  MarkerSize=10  GraphicType=FromGeometry  InertiaType=CalculateFromGeometry  Mass=1  MassUnits=kg  MomentsOfInertia=[1 1 1]  MomentsOfInertiaUnits=kg*m^2  PolygonNumSides=3  GraphicOpacity=1.0  PolygonOuterRadius=1  PolygonOuterRadiusUnits=m  ProductsOfInertia=[0 0 0]  ProductsOfInertiaUnits=kg*m^2  GraphicShininess=75  GraphicSpecularColor=[0.5 0.5 0.5 1.0]  GraphicVisPropType=SimpleVisualProperties
  Single Bracket : sm_backhoe_lib/Single Bracket  Hbracket=Lbase  Wbracket=Wbase  Tbracket=0.02  Hhole=Lbase-(Wbase/2)  Rhole=Rbp  Nc=circlePointsCylB  bracketColor=connColor  rho=rhoConn
      settings: SourceProductBaseCode=MS
  Base Hole : PMIOPort  Side=Right
  Prismatic : PMIOPort  Port=2  Side=Left
  connections:
  Single Bracket/RConn1 -- Base Hole/RConn1
  Single Bracket/LConn1 -- Base to Cylinder Transform/RConn1
  Base to Cylinder Transform/LConn1 -- Cylinder/RConn1
  Prismatic/RConn1 -- Cylinder/LConn1

== system sm_forklift/Forklift/Masts/Tilt Mechanism/Left Tilt Cylinder/Hydraulic Actuator ==
  Pressure Input : Inport
  Add : Sum
  Add1 : Sum  Inputs=+-
  Custom Hydraulic Fluid : fl_lib/Hydraulic/Hydraulic Utilities/Custom Hydraulic Fluid  density=850 kg/m^3  viscosity_kin=18e-6 m^2/s  bulk=0.8e9 Pa  alpha=0.005  range_error=2
      settings: SourceProductBaseCode=SS  InternalSimscapePortConfiguration="{\"Bottom\":[],\"Left\":[],\"Right\":[{\"id\":\"G\",\"label\":\"\",\"type\":\"foundation.hydraulic.hydraulic\"}],\"Top\":[]}"
  Cylinder Side Chamber : fl_lib/Hydraulic/Hydraulic Elements/Translational Hydro-Mechanical Converter  area=pi*(Rcyl^2) m^2  or=1  compressibility=0  displacement_spec=foundation.enum.DisplacementSpec.Calculate  init_pos=0 m  V_dead=1e-4 m^3  k_sh=1.4  initial_pressure=0 Pa
      settings: SourceProductBaseCode=SS  InternalSimscapePortConfiguration="{\"Bottom\":[],\"Left\":[{\"id\":\"C\",\"label\":\"C\",\"type\":\"foundation.mechanical.translational.translational\"},{\"id\":\"A\",\"label\":\"A\",\"type\":\"foundation.hydraulic.hydraulic\"}],\"Right\":[{\"id\":\"R\",\"label\":\"R\",\"type\":\"foundation.mechanical.translational.translational\"}],\"Top\":[]}"
  Gain : Gain  Gain=1/2
  Gain1 : Gain  Gain=1/2
  Hydraulic Reference : fl_lib/Hydraulic/Hydraulic Elements/Hydraulic Reference
  Linear Hydraulic Resistance : fl_lib/Hydraulic/Hydraulic Elements/Linear Hydraulic Resistance  resistance=1e5 Pa/(m^3/s)  q_specify=off  q_priority=None  q=0.001 m^3/s  q_nominal_specify=off  q_nominal_unit=m^3/s  q_nominal_value=1  p_specify=off  p_priority=None  p=0 Pa  p_nominal_specify=off  p_nominal_unit=Pa  p_nominal_value=1
      settings: SourceProductBaseCode=SS  InternalSimscapePortConfiguration="{\"Bottom\":[],\"Left\":[{\"id\":\"A\",\"label\":\"A\",\"type\":\"foundation.hydraulic.hydraulic\"}],\"Right\":[{\"id\":\"B\",\"label\":\"B\",\"type\":\"foundation.hydraulic.hydraulic\"}],\"Top\":[]}"
  Linear Hydraulic Resistance1 : fl_lib/Hydraulic/Hydraulic Elements/Linear Hydraulic Resistance  resistance=1e5 Pa/(m^3/s)  q_specify=off  q_priority=None  q=0.001 m^3/s  q_nominal_specify=off  q_nominal_unit=m^3/s  q_nominal_value=1  p_specify=off  p_priority=None  p=0 Pa  p_nominal_specify=off  p_nominal_unit=Pa  p_nominal_value=1
      settings: SourceProductBaseCode=SS  InternalSimscapePortConfiguration="{\"Bottom\":[],\"Left\":[{\"id\":\"A\",\"label\":\"A\",\"type\":\"foundation.hydraulic.hydraulic\"}],\"Right\":[{\"id\":\"B\",\"label\":\"B\",\"type\":\"foundation.hydraulic.hydraulic\"}],\"Top\":[]}"
  Mechanical Translational Reference : fl_lib/Mechanical/Translational Elements/Mechanical Translational Reference
  Nominal Pressure : Constant  Value=350
  Piston Head Side Chamber : fl_lib/Hydraulic/Hydraulic Elements/Translational Hydro-Mechanical Converter  area=pi*(Rcyl^2) m^2  or=2  compressibility=0  displacement_spec=foundation.enum.DisplacementSpec.Calculate  init_pos=0 m  V_dead=1e-4 m^3  k_sh=1.4  initial_pressure=0 Pa
      settings: SourceProductBaseCode=SS  InternalSimscapePortConfiguration="{\"Bottom\":[],\"Left\":[{\"id\":\"C\",\"label\":\"C\",\"type\":\"foundation.mechanical.translational.translational\"},{\"id\":\"A\",\"label\":\"A\",\"type\":\"foundation.hydraulic.hydraulic\"}],\"Right\":[{\"id\":\"R\",\"label\":\"R\",\"type\":\"foundation.mechanical.translational.translational\"}],\"Top\":[]}"
  Pressure Difference : fl_lib/Hydraulic/Hydraulic Sources/Hydraulic Pressure Source
      settings: SourceProductBaseCode=SS  InternalSimscapePortConfiguration="{\"Bottom\":[],\"Left\":[{\"id\":\"P\",\"label\":\"P\",\"type\":\"foundation.hydraulic.hydraulic\"}],\"Right\":[{\"id\":\"S\",\"label\":\"S\",\"type\":\"input\"},{\"id\":\"T\",\"label\":\"T\",\"type\":\"foundation.hydraulic.hydraulic\"}],\"Top\":[]}"
  Pressure Difference1 : fl_lib/Hydraulic/Hydraulic Sources/Hydraulic Pressure Source
      settings: SourceProductBaseCode=SS  InternalSimscapePortConfiguration="{\"Bottom\":[],\"Left\":[{\"id\":\"P\",\"label\":\"P\",\"type\":\"foundation.hydraulic.hydraulic\"}],\"Right\":[{\"id\":\"S\",\"label\":\"S\",\"type\":\"input\"},{\"id\":\"T\",\"label\":\"T\",\"type\":\"foundation.hydraulic.hydraulic\"}],\"Top\":[]}"
  Simulink-PS Converter : nesl_utility/Simulink-PS Converter  PhysicalDomain=network_engine_domain  SubClassName=ps_input  LeftPortType=input  RightPortType=output  PseudoPeriodic=off  Frequencies=[]  NoiseDistribution=none  NoiseParameters=[]  Unit=bar  AffineConversion=off  FilteringAndDerivatives=filter  SimscapeFilterOrder=1  InputFilterTimeConstant=.001  UdotUserProvided=1
      settings: SourceProductBaseCode=PW,SS
  Simulink-PS Converter1 : nesl_utility/Simulink-PS Converter  PhysicalDomain=network_engine_domain  SubClassName=ps_input  LeftPortType=input  RightPortType=output  PseudoPeriodic=off  Frequencies=[]  NoiseDistribution=none  NoiseParameters=[]  Unit=bar  AffineConversion=off  FilteringAndDerivatives=filter  SimscapeFilterOrder=1  InputFilterTimeConstant=.001  UdotUserProvided=1
      settings: SourceProductBaseCode=PW,SS
  R : PMIOPort  Side=Right
  C : PMIOPort  Port=2  Side=Right
  wires:
  Gain1/1 -> Add1/2
  Add1/1 -> Simulink-PS Converter1/1
  Add/1 -> Simulink-PS Converter/1
  Gain/1 -> Add/1
  Nominal Pressure/1 -> Add1/1, Add/2
  Pressure Input/1 -> Gain1/1, Gain/1
  connections:
  Linear Hydraulic Resistance1/LConn1 -- Pressure Difference1/LConn1
  Linear Hydraulic Resistance1/RConn1 -- Piston Head Side Chamber/LConn2
  Linear Hydraulic Resistance/RConn1 -- Cylinder Side Chamber/LConn2
  Simulink-PS Converter1/RConn1 -- Pressure Difference1/RConn1
  Simulink-PS Converter/RConn1 -- Pressure Difference/RConn1
  Pressure Difference1/RConn2 -- Pressure Difference/RConn2 -- Hydraulic Reference/LConn1
  Pressure Difference/LConn1 -- Linear Hydraulic Resistance/LConn1 -- Custom Hydraulic Fluid/RConn1
  R/RConn1 -- Piston Head Side Chamber/RConn1 -- Cylinder Side Chamber/RConn1
  Cylinder Side Chamber/LConn1 -- C/RConn1 -- Piston Head Side Chamber/LConn1 -- Mechanical Translational Reference/LConn1

== system sm_forklift/Forklift/Masts/Tilt Mechanism/Left Tilt Cylinder/Piston Assembly ==
  Piston : sm_lib/Body Elements/Cylindrical Solid  GraphicAmbientColor=[0.15 0.15 0.15 1.0]  BasedOnType=Density  CenterOfMass=[0 0 0]  CenterOfMassUnits=m  GraphicDiffuseColor=pistColor  CylinderLength=Lpist  CylinderLengthUnits=m  CylinderRadius=Rpist  CylinderRadiusUnits=m  Density=rhoPist  DensityUnits=kg/(m^3)  DoExposeReferenceFrame=on  GraphicEmissiveColor=[0.0 0.0 0.0 1.0]  ExportEntireGeometry=off  SerializedFrames=<Frames><Frame><Id>Frame1</Id><Value><Name>F1</Name><Origin><Source>GeometricFeature</Source><FeatureName>top surface</FeatureName></Origin><PrimaryAxis><DefinedDirection>+Z</DefinedDirection><Source>ReferenceFrame</Source><SourceDirection>+Z</SourceDirection><FeatureName></FeatureName></PrimaryAxis><SecondaryAxis><DefinedDirection>+X</DefinedDirection><Source>ReferenceFrame</Source><SourceDirection>+X</SourceDirection><FeatureName></FeatureName></SecondaryAxis></Value></Frame></Frames>  MarkerShape=Sphere  MarkerSize=10  GraphicType=FromGeometry  InertiaType=CalculateFromGeometry  Mass=1  MassUnits=kg  MomentsOfInertia=[1 1 1]  MomentsOfInertiaUnits=kg*m^2  GraphicOpacity=1.0  ProductsOfInertia=[0 0 0]  ProductsOfInertiaUnits=kg*m^2  GraphicShininess=75  GraphicSpecularColor=[0.5 0.5 0.5 1.0]  GraphicVisPropType=SimpleVisualProperties
  Piston to Head Transform : sm_lib/Frames and Transforms/Rigid Transform  TranslationMethod=StandardAxis  TranslationStandardOffset=Lpist/2  TranslationLengthUnit=m  TranslationStandardAxis=+Z  TranslationCartesianOffset=[0 0 0]  TranslationROffset=0  TranslationROffsetUnits=m  TranslationZOffset=0  TranslationZOffsetUnits=m  TranslationThetaOffset=0  TranslationThetaOffsetUnits=deg  RotationMethod=AlignedAxes  RotationAngleUnits=deg  RotationStandardAxis=-X  RotationAngle=90  RotationArbitraryAxis=[0 0 1]  FollAlignAxisA=+Y  BaseAlignAxisA=-Y  FollAlignAxisB=+Z  BaseAlignAxisB=+Z  RotationSequenceAxes=FollowerAxes  RotationSequence=XYX  RotationSequenceAngles=[0 0 0]  RotationSequenceAnglesUnits=deg  RotationMatrix=[1 0 0; 0 1 0; 0 0 1]
  Rigid Transform : sm_lib/Frames and Transforms/Rigid Transform  TranslationMethod=StandardAxis  TranslationStandardOffset=165  TranslationLengthUnit=mm  TranslationStandardAxis=-Z  TranslationCartesianOffset=[0 0 0]  TranslationROffset=0  TranslationROffsetUnits=m  TranslationZOffset=0  TranslationZOffsetUnits=m  TranslationThetaOffset=0  TranslationThetaOffsetUnits=deg  RotationMethod=None  RotationAngleUnits=deg  RotationStandardAxis=+Z  RotationAngle=0.0  RotationArbitraryAxis=[0 0 1]  FollAlignAxisA=+X  BaseAlignAxisA=+Y  FollAlignAxisB=+Y  BaseAlignAxisB=+Z  RotationSequenceAxes=FollowerAxes  RotationSequence=XYX  RotationSequenceAngles=[0 0 0]  RotationSequenceAnglesUnits=deg  RotationMatrix=[1 0 0; 0 1 0; 0 0 1]
  Single Bracket : sm_backhoe_lib/Single Bracket  Hbracket=Lhead  Wbracket=Whead  Tbracket=0.03  Hhole=Lhead-(Whead/2)  Rhole=Rhp  Nc=circlePointsPist  bracketColor=connColor  rho=rhoConn
      settings: SourceProductBaseCode=MS
  Prismatic : PMIOPort  Side=Left
  Head Hole : PMIOPort  Port=2  Side=Right
  connections:
  Single Bracket/RConn1 -- Head Hole/RConn1
  Piston to Head Transform/RConn1 -- Single Bracket/LConn1
  Piston to Head Transform/LConn1 -- Piston/RConn1
  Rigid Transform/RConn1 -- Prismatic/RConn1
  Piston/LConn1 -- Rigid Transform/LConn1

== system sm_forklift/Forklift/Masts/Tilt Mechanism/Left Tilt Cylinder/Simscape Interface ==
  Ideal Force Sensor : fl_lib/Mechanical/Mechanical Sensors/Ideal Force Sensor
  Ideal Translational Velocity Source : fl_lib/Mechanical/Mechanical Sources/Ideal Translational Velocity Source
  R : PMIOPort  Side=Right
  C : PMIOPort  Port=2  Side=Right
  F : PMIOPort  Port=3  Side=Left
  V : PMIOPort  Port=4  Side=Left
  connections:
  Ideal Force Sensor/RConn2 -- F/RConn1
  Ideal Force Sensor/LConn1 -- R/RConn1
  C/RConn1 -- Ideal Translational Velocity Source/RConn2
  V/RConn1 -- Ideal Translational Velocity Source/RConn1
  Ideal Force Sensor/RConn1 -- Ideal Translational Velocity Source/LConn1

== system sm_forklift/Forklift/Masts/Tilt Mechanism/Right Tilt Cylinder/Cylinder Assembly ==
  Base to Cylinder Transform : sm_lib/Frames and Transforms/Rigid Transform  TranslationMethod=StandardAxis  TranslationStandardOffset=(Lcyl/2)  TranslationLengthUnit=m  TranslationStandardAxis=-Z  TranslationCartesianOffset=[0 0 0]  TranslationROffset=0  TranslationROffsetUnits=m  TranslationZOffset=0  TranslationZOffsetUnits=m  TranslationThetaOffset=0  TranslationThetaOffsetUnits=deg  RotationMethod=AlignedAxes  RotationAngleUnits=deg  RotationStandardAxis=+X  RotationAngle=90  RotationArbitraryAxis=[0 0 1]  FollAlignAxisA=+X  BaseAlignAxisA=+X  FollAlignAxisB=+Z  BaseAlignAxisB=-Z  RotationSequenceAxes=FollowerAxes  RotationSequence=XYX  RotationSequenceAngles=[0 0 0]  RotationSequenceAnglesUnits=deg  RotationMatrix=[1 0 0; 0 1 0; 0 0 1]
  Cylinder : sm_lib/Body Elements/Extruded Solid  GraphicAmbientColor=[0.15 0.15 0.15 1.0]  BasedOnType=Density  CenterOfMass=[0 0 0]  CenterOfMassUnits=m  GraphicDiffuseColor=cylColor  ExportConvexHullGeometry=off  ExtrusionCrossSection=cylSection  ExtrusionCrossSectionUnits=m  Density=rhoCyl  DensityUnits=kg/(m^3)  DoExposeReferenceFrame=on  GraphicEmissiveColor=[0.0 0.0 0.0 1.0]  ExportEntireGeometry=off  ExtrusionLength=Lcyl  ExtrusionLengthUnits=m  ExtrusionType=General  SerializedFrames=<Frames><Frame><Id>Frame1</Id><Value><Name>F1</Name><Origin><Source>GeometricFeature</Source><FeatureName>top surface</FeatureName></Origin><PrimaryAxis><DefinedDirection>+Z</DefinedDirection><Source>ReferenceFrame</Source><SourceDirection>+Z</SourceDirection><FeatureName></FeatureName></PrimaryAxis><SecondaryAxis><DefinedDirection>+X</DefinedDirection><Source>ReferenceFrame</Source><SourceDirection>+X</SourceDirection><FeatureName></FeatureName></SecondaryAxis></Value></Frame></Frames>  MarkerShape=Sphere  MarkerSize=10  GraphicType=FromGeometry  InertiaType=CalculateFromGeometry  Mass=1  MassUnits=kg  MomentsOfInertia=[1 1 1]  MomentsOfInertiaUnits=kg*m^2  PolygonNumSides=3  GraphicOpacity=1.0  PolygonOuterRadius=1  PolygonOuterRadiusUnits=m  ProductsOfInertia=[0 0 0]  ProductsOfInertiaUnits=kg*m^2  GraphicShininess=75  GraphicSpecularColor=[0.5 0.5 0.5 1.0]  GraphicVisPropType=SimpleVisualProperties
  Single Bracket : sm_backhoe_lib/Single Bracket  Hbracket=Lbase  Wbracket=Wbase  Tbracket=0.02  Hhole=Lbase-(Wbase/2)  Rhole=Rbp  Nc=circlePointsCylB  bracketColor=connColor  rho=rhoConn
      settings: SourceProductBaseCode=MS
  Base Hole : PMIOPort  Side=Right
  Prismatic : PMIOPort  Port=2  Side=Left
  connections:
  Prismatic/RConn1 -- Cylinder/LConn1
  Base to Cylinder Transform/LConn1 -- Cylinder/RConn1
  Single Bracket/LConn1 -- Base to Cylinder Transform/RConn1
  Single Bracket/RConn1 -- Base Hole/RConn1

== system sm_forklift/Forklift/Masts/Tilt Mechanism/Right Tilt Cylinder/Piston Assembly ==
  Piston : sm_lib/Body Elements/Cylindrical Solid  GraphicAmbientColor=[0.15 0.15 0.15 1.0]  BasedOnType=Density  CenterOfMass=[0 0 0]  CenterOfMassUnits=m  GraphicDiffuseColor=pistColor  CylinderLength=Lpist  CylinderLengthUnits=m  CylinderRadius=Rpist  CylinderRadiusUnits=m  Density=rhoPist  DensityUnits=kg/(m^3)  DoExposeReferenceFrame=on  GraphicEmissiveColor=[0.0 0.0 0.0 1.0]  ExportEntireGeometry=off  SerializedFrames=<Frames><Frame><Id>Frame1</Id><Value><Name>F1</Name><Origin><Source>GeometricFeature</Source><FeatureName>top surface</FeatureName></Origin><PrimaryAxis><DefinedDirection>+Z</DefinedDirection><Source>ReferenceFrame</Source><SourceDirection>+Z</SourceDirection><FeatureName></FeatureName></PrimaryAxis><SecondaryAxis><DefinedDirection>+X</DefinedDirection><Source>ReferenceFrame</Source><SourceDirection>+X</SourceDirection><FeatureName></FeatureName></SecondaryAxis></Value></Frame></Frames>  MarkerShape=Sphere  MarkerSize=10  GraphicType=FromGeometry  InertiaType=CalculateFromGeometry  Mass=1  MassUnits=kg  MomentsOfInertia=[1 1 1]  MomentsOfInertiaUnits=kg*m^2  GraphicOpacity=1.0  ProductsOfInertia=[0 0 0]  ProductsOfInertiaUnits=kg*m^2  GraphicShininess=75  GraphicSpecularColor=[0.5 0.5 0.5 1.0]  GraphicVisPropType=SimpleVisualProperties
  Piston to Head Transform : sm_lib/Frames and Transforms/Rigid Transform  TranslationMethod=StandardAxis  TranslationStandardOffset=Lpist/2  TranslationLengthUnit=m  TranslationStandardAxis=+Z  TranslationCartesianOffset=[0 0 0]  TranslationROffset=0  TranslationROffsetUnits=m  TranslationZOffset=0  TranslationZOffsetUnits=m  TranslationThetaOffset=0  TranslationThetaOffsetUnits=deg  RotationMethod=AlignedAxes  RotationAngleUnits=deg  RotationStandardAxis=-X  RotationAngle=90  RotationArbitraryAxis=[0 0 1]  FollAlignAxisA=+Y  BaseAlignAxisA=-Y  FollAlignAxisB=+Z  BaseAlignAxisB=+Z  RotationSequenceAxes=FollowerAxes  RotationSequence=XYX  RotationSequenceAngles=[0 0 0]  RotationSequenceAnglesUnits=deg  RotationMatrix=[1 0 0; 0 1 0; 0 0 1]
  Rigid Transform : sm_lib/Frames and Transforms/Rigid Transform  TranslationMethod=StandardAxis  TranslationStandardOffset=165  TranslationLengthUnit=mm  TranslationStandardAxis=-Z  TranslationCartesianOffset=[0 0 0]  TranslationROffset=0  TranslationROffsetUnits=m  TranslationZOffset=0  TranslationZOffsetUnits=m  TranslationThetaOffset=0  TranslationThetaOffsetUnits=deg  RotationMethod=None  RotationAngleUnits=deg  RotationStandardAxis=+Z  RotationAngle=0.0  RotationArbitraryAxis=[0 0 1]  FollAlignAxisA=+X  BaseAlignAxisA=+Y  FollAlignAxisB=+Y  BaseAlignAxisB=+Z  RotationSequenceAxes=FollowerAxes  RotationSequence=XYX  RotationSequenceAngles=[0 0 0]  RotationSequenceAnglesUnits=deg  RotationMatrix=[1 0 0; 0 1 0; 0 0 1]
  Single Bracket : sm_backhoe_lib/Single Bracket  Hbracket=Lhead  Wbracket=Whead  Tbracket=0.03  Hhole=Lhead-(Whead/2)  Rhole=Rhp  Nc=circlePointsPist  bracketColor=connColor  rho=rhoConn
      settings: SourceProductBaseCode=MS
  Prismatic : PMIOPort  Side=Left
  Head Hole : PMIOPort  Port=2  Side=Right
  connections:
  Piston/LConn1 -- Rigid Transform/LConn1
  Rigid Transform/RConn1 -- Prismatic/RConn1
  Piston to Head Transform/LConn1 -- Piston/RConn1
  Piston to Head Transform/RConn1 -- Single Bracket/LConn1
  Single Bracket/RConn1 -- Head Hole/RConn1

== system sm_forklift/Warehouse/Racks/Rack 1/Palettes_1/Palette_800x1200_10_RIGID ==
  ReferenceFrame : sm_lib/Frames and Transforms/Reference Frame
  Solid : sm_lib/Body Elements/File Solid  ExtGeomFileName=Palette_800x1200.step  UnitType=FromFile  ExtGeomFileUnits=m  StepReaderType=HEX  ExportConvexHullGeometry=off  InertiaType=Custom  Mass=smiData.Solid(1).mass  MassUnits=kg  CenterOfMass=smiData.Solid(1).CoM  CenterOfMassUnits=m  MomentsOfInertia=smiData.Solid(1).MoI  MomentsOfInertiaUnits=kg*m^2  ProductsOfInertia=smiData.Solid(1).PoI  ProductsOfInertiaUnits=kg*m^2  BasedOnType=Density  Density=1000  DensityUnits=kg/m^3  DoExposeReferenceFrame=on  SerializedFrames=<Frames/>  GraphicType=FromGeometry  MarkerShape=Sphere  MarkerSize=10  GraphicVisPropType=SimpleVisualProperties  GraphicDiffuseColor=smiData.Solid(1).color  GraphicSpecularColor=[0.5 0.5 0.5 1.0]  GraphicAmbientColor=[0.15 0.15 0.15 1.0]  GraphicEmissiveColor=[0.0 0.0 0.0 1.0]  GraphicShininess=75  GraphicOpacity=smiData.Solid(1).opacity
  F : PMIOPort  Side=Left
  connections:
  Solid/RConn1 -- ReferenceFrame/RConn1 -- F/RConn1

== system sm_forklift/Warehouse/Racks/Rack 1/Palettes_1/Palette_800x1200_11_RIGID ==
  ReferenceFrame : sm_lib/Frames and Transforms/Reference Frame
  Solid : sm_lib/Body Elements/File Solid  ExtGeomFileName=Palette_800x1200.step  UnitType=FromFile  ExtGeomFileUnits=m  StepReaderType=HEX  ExportConvexHullGeometry=off  InertiaType=Custom  Mass=smiData.Solid(1).mass  MassUnits=kg  CenterOfMass=smiData.Solid(1).CoM  CenterOfMassUnits=m  MomentsOfInertia=smiData.Solid(1).MoI  MomentsOfInertiaUnits=kg*m^2  ProductsOfInertia=smiData.Solid(1).PoI  ProductsOfInertiaUnits=kg*m^2  BasedOnType=Density  Density=1000  DensityUnits=kg/m^3  DoExposeReferenceFrame=on  SerializedFrames=<Frames/>  GraphicType=FromGeometry  MarkerShape=Sphere  MarkerSize=10  GraphicVisPropType=SimpleVisualProperties  GraphicDiffuseColor=smiData.Solid(1).color  GraphicSpecularColor=[0.5 0.5 0.5 1.0]  GraphicAmbientColor=[0.15 0.15 0.15 1.0]  GraphicEmissiveColor=[0.0 0.0 0.0 1.0]  GraphicShininess=75  GraphicOpacity=smiData.Solid(1).opacity
  F : PMIOPort  Side=Left
  connections:
  Solid/RConn1 -- ReferenceFrame/RConn1 -- F/RConn1
